simulink model "t1_it2_fis_comp"  (R2023a)
settings: Solver=VariableStepAuto  StartTime=0.0  StopTime=10.0  RelTol=1e-3
libraries: fuzblock x2
settings Model: Creator=yingb  LastModifiedBy=yingb

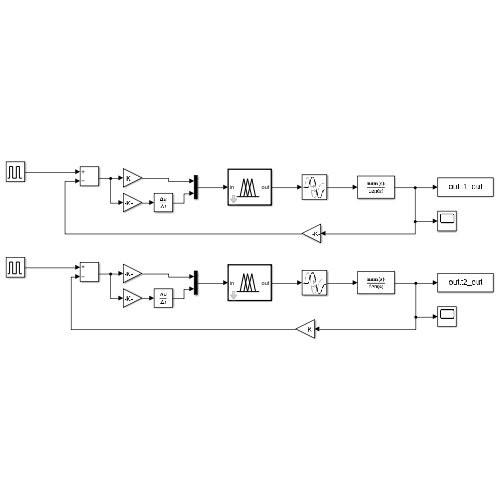
[thumbnail: Simulink's stored preview of the top-level diagram]
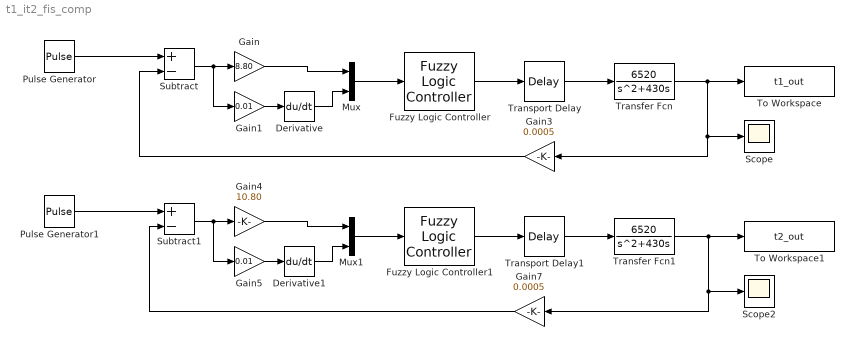
== system t1_it2_fis_comp ==
  Derivative : Derivative
  Derivative1 : Derivative
  Fuzzy Logic Controller : fuzblock/Fuzzy Logic  Controller  FIS='type1_fis.fis'  OutputSampleNumber=101  DataType=double  FuzzifiedInputs=off  RuleFiringStrengths=off  RuleOutputs=off  AggregatedOutputs=off  SimulateUsing=Interpreted execution  OutOfRangeInputValueMessage=warning  NoRuleFiredMessage=warning  EmptyOutputFuzzySetMessage=warning
  Fuzzy Logic Controller1 : fuzblock/Fuzzy Logic  Controller  FIS='itype2_fis.fis'  OutputSampleNumber=101  DataType=double  FuzzifiedInputs=off  RuleFiringStrengths=off  RuleOutputs=off  AggregatedOutputs=off  SimulateUsing=Interpreted execution  OutOfRangeInputValueMessage=warning  NoRuleFiredMessage=warning  EmptyOutputFuzzySetMessage=warning
  Gain : Gain  Gain=8.80
  Gain1 : Gain  Gain=0.01  OutMin=[-0.15]  OutMax=[0.15]
  Gain3 : Gain  Gain=0.0005
  Gain4 : Gain  Gain=10.80
  Gain5 : Gain  Gain=0.01  OutMin=[-0.15]  OutMax=[0.15]
  Gain7 : Gain  Gain=0.0005
  Mux : Mux  Inputs=2
  Mux1 : Mux  Inputs=2
  Pulse Generator : DiscretePulseGenerator  PulseType=Time based  Amplitude=0.3  Period=4  PulseWidth=50
  Pulse Generator1 : DiscretePulseGenerator  PulseType=Time based  Amplitude=0.3  Period=4  PulseWidth=50
  Scope : Scope
      settings: Tag=t1_fis
  Scope2 : Scope
      settings: Tag=t1_fis
  Subtract : Sum  Inputs=+-
  Subtract1 : Sum  Inputs=+-
  To Workspace : ToWorkspace  VariableName=t1_out  SaveFormat=Timeseries  SampleTime=0.005
  To Workspace1 : ToWorkspace  VariableName=t2_out  SaveFormat=Timeseries  SampleTime=0.005
  Transfer Fcn : TransferFcn  Numerator=[6520]  Denominator=[1 430 0]  ParameterTunability=Optimized
  Transfer Fcn1 : TransferFcn  Numerator=[6520]  Denominator=[1 430 0]  ParameterTunability=Optimized
  Transport Delay : TransportDelay  DelayTime=0.005
  Transport Delay1 : TransportDelay  DelayTime=0.005
  wires:
  Subtract/1 -> Gain1/1, Gain/1
  Transfer Fcn/1 -> To Workspace/1, Scope/1, Gain3/1
  Gain/1 -> Mux/1
  Derivative/1 -> Mux/2
  Transport Delay/1 -> Transfer Fcn/1
  Gain1/1 -> Derivative/1
  Gain3/1 -> Subtract/2
  Pulse Generator/1 -> Subtract/1
  Gain7/1 -> Subtract1/2
  Transport Delay1/1 -> Transfer Fcn1/1
  Gain5/1 -> Derivative1/1
  Subtract1/1 -> Gain5/1, Gain4/1
  Transfer Fcn1/1 -> To Workspace1/1, Scope2/1, Gain7/1
  Gain4/1 -> Mux1/1
  Pulse Generator1/1 -> Subtract1/1
  Derivative1/1 -> Mux1/2
  Mux/1 -> Fuzzy Logic Controller/1
  Fuzzy Logic Controller/1 -> Transport Delay/1
  Mux1/1 -> Fuzzy Logic Controller1/1
  Fuzzy Logic Controller1/1 -> Transport Delay1/1
